simulink model "wrapping_example"  (R2019b)
settings: Solver=VariableStepAuto  StartTime=0.0  StopTime=10.0  RelTol=1e-3
settings Model: Creator=szgno  LastModifiedBy=szgno

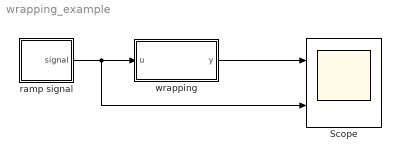
== system wrapping_example ==
  Scope : Scope  NumInputPorts=2
  ramp signal : Subsystem
  wrapping : Subsystem  mask{u_max=360}
      mask prompts: u_max "Maximum Wrapping Range"
      mask Display:
      | pos = get_param(gcb,'Position')
      | width = pos(3)-pos(1); % right-left
      | height = pos(4)-pos(2); % top-bottom
      | x = (0.1*width):0.01:(0.9*width);
      | plot(x,mod(x,width/3.5)-width/7+height/2)
  wires:
  wrapping/1(y) -> Scope/1
  ramp signal/1(signal) -> Scope/2, wrapping/1(u)

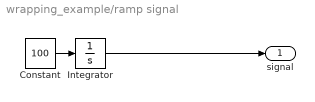
== system wrapping_example/ramp signal ==
  Constant : Constant  Value=100  SampleTime=0.01
  Integrator : Integrator
  signal : Outport
  wires:
  Constant/1 -> Integrator/1
  Integrator/1 -> signal/1

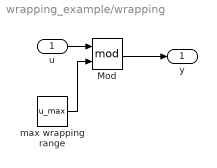
== system wrapping_example/wrapping ==
  u : Inport
  Mod : Math  Operator=mod  SaturateOnIntegerOverflow=on
  max wrapping range : Constant  Value=u_max
  y : Outport
  wires:
  max wrapping range/1 -> Mod/2
  u/1 -> Mod/1
  Mod/1 -> y/1
